simulink model "active_quartersusp"  (R2019a)
settings: Solver=VariableStepAuto  StartTime=0.0  StopTime=10.0  RelTol=1e-5
settings Model: Creator=dağlar  LastModifiedBy=dağlar

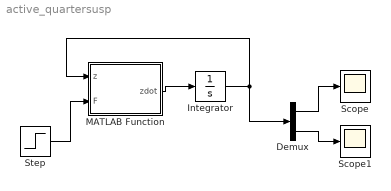
== system active_quartersusp ==
  Demux : Demux  Outputs=2
  Integrator : Integrator  InitialCondition=[0;0;0;0]
  MATLAB Function : MATLAB Function  TreatAsAtomicUnit=on
  Scope : Scope
  Scope1 : Scope
  Step : Step  SampleTime=0
  wires:
  MATLAB Function/1(zdot) -> Integrator/1
  Integrator/1 -> MATLAB Function/1(z), Demux/1
  Demux/1 -> Scope/1
  Demux/2 -> Scope1/1
  Step/1 -> MATLAB Function/2(F)

== matlab function active_quartersusp/MATLAB Function ==
  data: z input; zdot output; F input
function zdot = fcn(z,F)
m1 = 300;
m2 = 60;
k1 = 16000;
k2 = 19000;
b1 = 1000;
b2 = 1000;


A=[0 1 0 0; 
  -k1/m1 -b1/m1 k1/m1 b1/m1;
  0 0 0 1;
  k1/m2 b1/m2 (-k1-k2)/m2 (-b1-b2)/m2];

B=[0;
   1/m1;
   0;
   1/m2];




zdot = A*z+ B*F;
end
